simulink model "ACTUAL_REV3_TESTMETHOD"  (R2025b)
settings: Solver=FixedStepAuto  StartTime=0.0  StopTime=inf  RelTol=1e-3
undefined symbols (not defined in the file): IO397, Pull, pull, up
libraries: speedgoatlib_IO613 x3, speedgoatlib_fpga_analog_io x2, canmsglib x2, speedgoatlib_fpga x1
settings Model: Creator=liamb  LastModifiedBy=maxbr
settings SolverCC: ConcurrentTasks=on  PositivePriorityOrder=on
settings OptimizationCC: BlockReduction=off  OptimizeBlockIOStorage=off
settings DebuggingCC: TasksWithSamePriorityMsg=none
settings HardwareCC: ProdBitPerLong=64.0  ProdLongLongMode=on  ProdHWDeviceType=Intel->x86-64 (Linux 64)
settings RTWCC: SystemTargetFile=speedgoat.tlc  TemplateMakefile=slrealtime_default_tmf  Toolchain=Simulink Real-Time Toolchain  BuildConfiguration=Faster Runs  CodeExecutionProfiling=on  TargetLang=C++  Description=Speedgoat Real-Time Target Machine
settings SimulinkRealTimeTargetCC: SLRTFileLogMaxRuns=1.0  ExtModeMaxTrigDuration=10.0  ExtModeStaticAllocSize=1000000.0  ExtModeTransport=0.0  MultiwordLength=2048.0  DynamicStringBufferSize=256.0  PreserveMATLABNamespacesInGeneratedCode=on  SubcomponentCodeInterfacePackaging=Reusable function  MATLABClassNameForMDSCustomization=Simulink.SoftwareTarget.GRTCustomization  InstructionSetFMA=off  LogToMDFFile=off

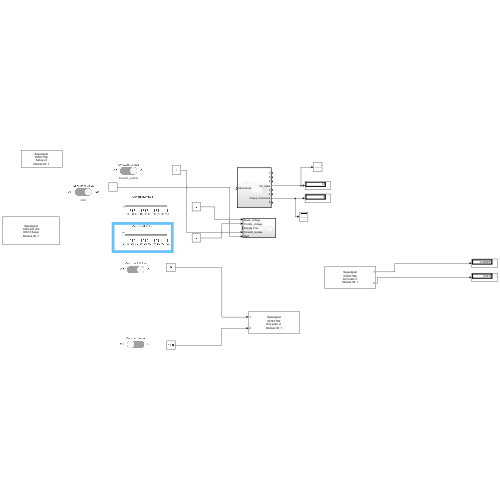
[thumbnail: Simulink's stored preview of the top-level diagram]
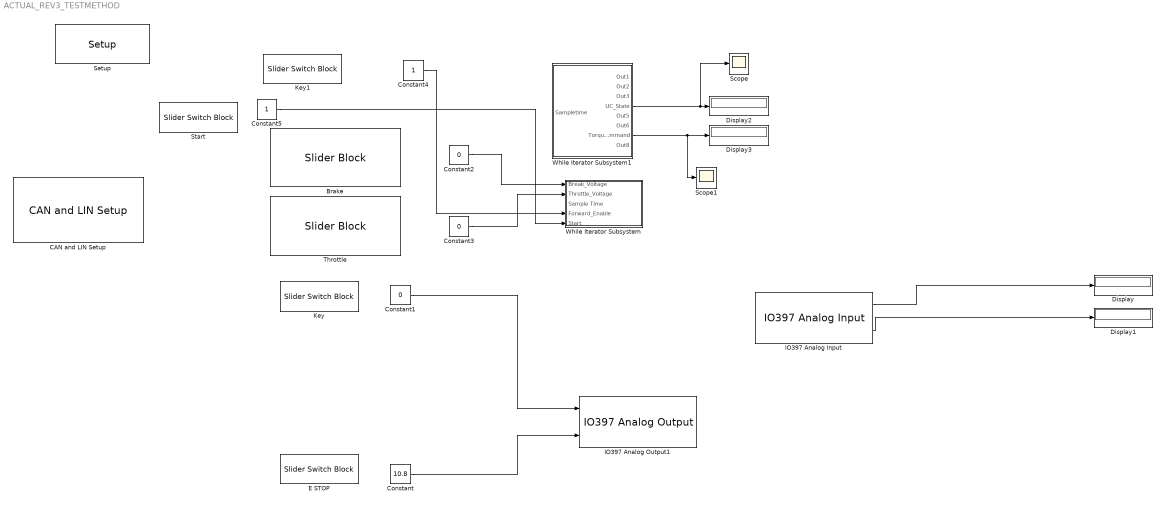
== system ACTUAL_REV3_TESTMETHOD ==
  Brake : SliderBlock
  "CAN and LIN Setup " : speedgoatlib_IO613/CAN and LIN Setup   moduleInitValues="[613    1    1   -1   -1]"  id=1  moduleType=IO613  pciSlot=-1  canChn1=CAN (HS)  canChn2=CAN (HS)  canChn3=Disabled  canChn4=Disabled  linChn1=Disabled  linChn2=Disabled  canInitStructArray=[]  canTermStructArray=[]  canChn1InitValues="[2   4   1  31   8   2   1  15   4]"  arbBdrChn1=500 kBaud  arbManBdrChn1=[4,1,31,8]  fdBdrChn1=2.0 MBaud  fdManBdrChn1=[2,1,15,4]  canChn2InitValues="[2   4   1  31   8   2   1  15   4]"  arbBdrChn2=500 kBaud  arbManBdrChn2=[4,1,31,8]  fdBdrChn2=2.0 MBaud  fdManBdrChn2=[2,1,15,4]  canChn3InitValues="[1   2   1  31   8   2   1   5   2]"  arbBdrChn3=1.0 MBaud  arbManBdrChn3=[2,1,31,8]  fdBdrChn3=5.0 MBaud  fdManBdrChn3=[2,1,5,2]  canChn4InitValues="[1   2   1  31   8   2   1   5   2]"  arbBdrChn4=1.0 MBaud  arbManBdrChn4=[2,1,31,8]  fdBdrChn4=5.0 MBaud  fdManBdrChn4=[2,1,5,2]  bdrLIN1=19200  linChn1InitValues="[1  19200]"  bdrLIN2=19200  linChn2InitValues="[1  19200]"
      settings: LibrarySourceBlock=speedgoatlib_CANLIN_OfA2/CAN and LIN Setup
  Constant : Constant  Value=10.8
  Constant1 : Constant  Value=0
  Constant2 : Constant  Value=0
  Constant3 : Constant  Value=0
  Constant4 : Constant
  Constant5 : Constant
  Display{,1..3} (4 alike) : Display
  E STOP : SliderSwitchBlock
  IO397 Analog Input : speedgoatlib_fpga_analog_io/IO397/IO397 Analog Input  openMaskCallback=0  id=1  chan=[1,2]  range=+5.12 V  parAiTriggerMode=I/O Module Clock  parAiInternalSignal=None  parAiDioTriggerChannel=1  parAiSampleRate=0  trigger=Initiator  ts=0.001
      settings: SourceProductName=Analog IO
  IO397 Analog Output1 : speedgoatlib_fpga_analog_io/IO397/IO397 Analog Output  id=1  chan=[1,2]  initVal=0  resetVal=0  ts=0.001  span=+-10.8 V
      settings: SourceProductName=Analog IO
  Key : SliderSwitchBlock
  Key1 : SliderSwitchBlock
      settings: AttributesFormatString=forward_enable
  Scope : Scope
      settings: ActiveDisplayYMinimum=-1  ActiveDisplayYMaximum=1
  Scope1 : Scope
      settings: ActiveDisplayYMinimum=-1  ActiveDisplayYMaximum=1
  Setup : speedgoatlib_fpga/Setup/Setup  board=IO397-50k  id=1  pciSlot=-1  device_id=1  bitstreamFilePath=C:\ProgramData\Speedgoat\bitstreams\io_configuration_package\R2025b\io397  bitstreamFile=speedgoat_IO397_HIL.mat  fpgaFreq=75000000  enableDma=off  rearEnb_1=off  rearIO_1=None  rearEnb_2=off  rearIO_2=None  ProgSpiFlash=off  ProgBPIFlash=off  useFpgaDmaController=off  dmaStopOnOverload=on  dmaModeSequential=on  dmaModeParallel=off  dmaTrigFixTime=on  dmaTrigA2B=off  dmaTriggerSourceSel=0  PullRPort15=pull-up 3.3V  PullRPort31=pull-up 3.3V  PullRPort47=pull-up 3.3V  PullRPort63=pull-up 3.3V  diffLineTermination_1=on  diffLineTermination_2=on  diffLineTermination_3=on  diffLineTermination_4=on  diffLineTermination_5=on  diffLineTermination_6=on  diffLineTermination_7=on  diffLineTermination_8=on  diffLineTermination_9=on  diffLineTermination_10=on  diffLineTermination_11=on  diffLineTermination_12=on  diffLineTermination_13=on  diffLineTermination_14=on  diffLineTermination_15=on  diffLineTermination_16=on  diffLineTermination_17=on  diffLineTermination_18=on  diffLineTermination_19=on  diffLineTermination_20=on  diffLineTermination_21=on  diffLineTermination_22=on  diffLineTermination_23=on  diffLineTermination_24=on  diffLineTermination_25=on  diffLineTermination_26=on  diffLineTermination_27=on  diffLineTermination_28=on  diffLineTermination_29=on  diffLineTermination_30=on  diffLineTermination_31=on  diffLineTermination_32=on  ioVoltageDropDown1=3.3V  pullResistorDropDown1_1=Pull-up  pullResistorDropDown1_2=Pull-up  pullResistorDropDown1_3=Pull-up  pullResistorDropDown1_4=Pull-up  pullResistorDropDown1_5=Pull-up  pullResistorDropDown1_6=Pull-up  pullResistorDropDown1_7=Pull-up  pullResistorDropDown1_8=Pull-up  ttlIsImplementedCheckBox1=off  pullResistorDropDown2=Pull-up  ioVoltageDropDown2=3.3V  ttlIsImplementedCheckBox2=off  pullResistorDropDown3=Pull-up  ioVoltageDropDown3=3.3V  ttlIsImplementedCheckBox3=off  pullResistorDropDown4=Pull-up  ioVoltageDropDown4=3.3V  ttlIsImplementedCheckBox4=off  pullResistorDropDown5=Pull-up  ioVoltageDropDown5=3.3V  ttlIsImplementedCheckBox5=off  pullResistorDropDown6=Pull-up  ioVoltageDropDown6=3.3V  ttlIsImplementedCheckBox6=off  pullResistorDropDown7=Pull-up  ioVoltageDropDown7=3.3V  ttlIsImplementedCheckBox7=off  pullResistorDropDown8=Pull-up  ioVoltageDropDown8=3.3V  ttlIsImplementedCheckBox8=off  terminationCheckBox1=off  terminationCheckBox2=off  terminationCheckBox3=off  terminationCheckBox4=off  diffIsImplementedCheckBox1=off  terminationCheckBox5=off  terminationCheckBox6=off  terminationCheckBox7=off  terminationCheckBox8=off  diffIsImplementedCheckBox2=off  terminationCheckBox9=off  terminationCheckBox10=off  terminationCheckBox11=off  terminationCheckBox12=off  diffIsImplementedCheckBox3=off  terminationCheckBox13=off  terminationCheckBox14=off  terminationCheckBox15=off  terminationCheckBox16=off  diffIsImplementedCheckBox4=off  terminationCheckBox17=off  terminationCheckBox18=off  terminationCheckBox19=off  terminationCheckBox20=off  diffIsImplementedCheckBox5=off  terminationCheckBox21=off  terminationCheckBox22=off  terminationCheckBox23=off  terminationCheckBox24=off  diffIsImplementedCheckBox6=off  terminationCheckBox25=off  terminationCheckBox26=off  terminationCheckBox27=off  terminationCheckBox28=off  diffIsImplementedCheckBox7=off  terminationCheckBox29=off  terminationCheckBox30=off  terminationCheckBox31=off  terminationCheckBox32=off  diffIsImplementedCheckBox8=off  PullRPort0_1=pull-up  VioPort0_1=3.3V  PullRPort1_1=pull-up  VioPort1_1=3.3V  PullRPort2_1=pull-up  VioPort2_1=3.3V  PullRPort3_1=pull-up  VioPort3_1=3.3V  PullRPort4_1=pull-up  VioPort4_1=3.3V  PullRPort5_1=pull-up  VioPort5_1=3.3V  PullRPort6_1=pull-up  VioPort6_1=3.3V  diffLineTermination_rear1_1=on  diffLineTermination_rear1_2=on  diffLineTermination_rear1_3=on  diffLineTermination_rear1_4=on  diffLineTermination_rear1_5=on  diffLineTermination_rear1_6=on  diffLineTermination_rear1_7=on  diffLineTermination_rear1_8=on  PullRPort0_2=pull-up  VioPort0_2=3.3V  PullRPort1_2=pull-up  VioPort1_2=3.3V  PullRPort2_2=pull-up  VioPort2_2=3.3V  PullRPort3_2=pull-up  VioPort3_2=3.3V  PullRPort4_2=pull-up  VioPort4_2=3.3V  PullRPort5_2=pull-up  VioPort5_2=3.3V  PullRPort6_2=pull-up  VioPort6_2=3.3V  diffLineTermination_rear2_1=on  diffLineTermination_rear2_2=on  diffLineTermination_rear2_3=on  diffLineTermination_rear2_4=on  diffLineTermination_rear2_5=on  diffLineTermination_rear2_6=on  diffLineTermination_rear2_7=on  diffLineTermination_rear2_8=on
      settings: SourceProductName=IO3xx
  Start : SliderSwitchBlock
      settings: AttributesFormatString=start
  Throttle : SliderBlock
  While Iterator Subsystem : Subsystem  TreatAsAtomicUnit=on
  While Iterator Subsystem1 : Subsystem  TreatAsAtomicUnit=on
  wires:
  Constant1/1 -> IO397 Analog Output1/1
  Constant3/1 -> While Iterator Subsystem/2(Throttle_Voltage)
  Constant2/1 -> While Iterator Subsystem/1(Break_Voltage)
  Constant/1 -> IO397 Analog Output1/2
  IO397 Analog Input/1 -> Display/1
  IO397 Analog Input/2 -> Display1/1
  While Iterator Subsystem1/7(Torque_Command) -> Scope1/1, Display3/1
  While Iterator Subsystem1/4(UC_State) -> Scope/1, Display2/1
  Constant4/1 -> While Iterator Subsystem/4(Forward_Enable)
  Constant5/1 -> While Iterator Subsystem/5(Start)

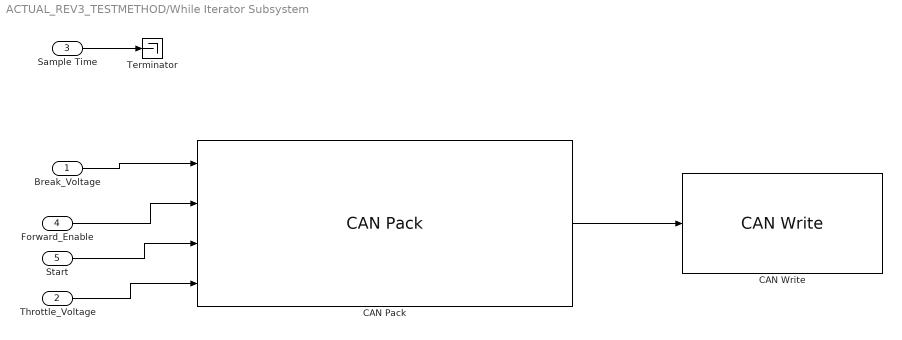
== system ACTUAL_REV3_TESTMETHOD/While Iterator Subsystem ==
  Break_Voltage : Inport
  Throttle_Voltage : Inport  Port=2
  Sample Time : Inport  Port=3
  Forward_Enable : Inport  Port=4
  Start : Inport  Port=5
  CAN Pack : canmsglib/CAN Pack  CANdbFile=C:\Users\maxbr\OneDrive\Documents\updatedpowertraindbcusethis.dbc  MsgList=Throttle_Position_and_Errors  MsgName=Throttle_Position_and_Errors  MsgIDType=Standard (11-bit identifier)  MsgIdentifier=208  CANIDInput=off  MsgLength=8  Remote=off  ApplyMinMax=off  BusOutput=off  SignalInfo={'Break_Voltage','16','16','LE','unsigned','Standard','0','1','0','0','65535';'Forward_Enable','48','1','LE','unsigned','Standard','0','1','0','0','1';'Start','49','1','LE','unsigned','Standard','0','1','0','0','1';'Throttle_Voltage','0','16','LE','unsigned','Standard','0','1','0','0','65535'}
      settings: DataFormat=CANdb specified signals
  "CAN Write " : speedgoatlib_IO613/CAN Write   moduleType=IO613  id=1  channel=1  canType=CAN (HS)  useBusIn=off  numOfMsg=1  enableInput=off  enableStatusPort=off  initValues=[613 1 0.01 0 1 1 0 1 0 0]  ts=.01
      settings: SourceProductName=IO613
  Terminator : Terminator
  wires:
  Break_Voltage/1 -> CAN Pack/1
  CAN Pack/1 -> "CAN Write "/1
  Sample Time/1 -> Terminator/1
  Forward_Enable/1 -> CAN Pack/2
  Throttle_Voltage/1 -> CAN Pack/4
  Start/1 -> CAN Pack/3

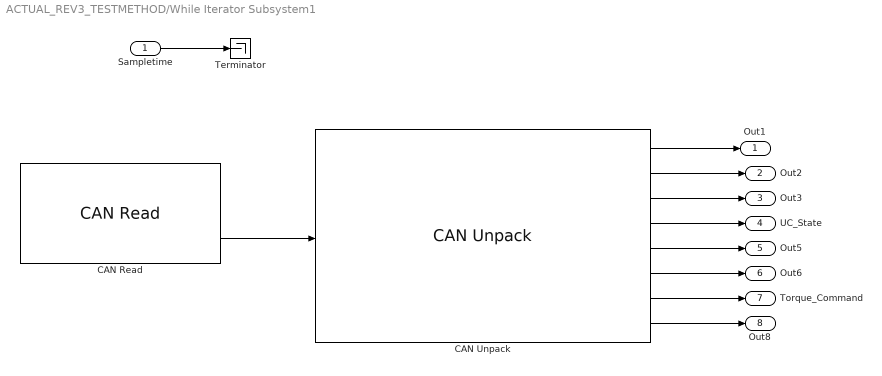
== system ACTUAL_REV3_TESTMETHOD/While Iterator Subsystem1 ==
  Sampletime : Inport
  "CAN Read " : speedgoatlib_IO613/CAN Read   moduleType=IO613  id=1  channel=1  canType=CAN (HS)  useBusOut=off  HasMulRead=Single Read from Buffer (FIFO)  MsgIDlist=[1 2]  isEFF=off  LabelInHex=on  enableInput=off  ts=.01  initValues=[613 1 0.01 0 1 1 0 0 0 1 2 1 2]
      settings: SourceProductName=IO613
  CAN Unpack : canmsglib/CAN Unpack  CANdbFile=C:\Users\maxbr\OneDrive\Documents\updatedpowertraindbcusethis.dbc  MsgList=M192_Command_Message  MsgName=M192_Command_Message  MsgIDType=Standard (11-bit identifier)  MsgIdentifier=192  MsgLength=8  SignalInfo={'VCU_INV_Direction_Command','32','1','LE','unsigned','Standard','0','1','0','0','1';'VCU_INV_Inverter_Discharge','41','1','LE','unsigned','Standard','0','1','0','0','1';'VCU_INV_Inverter_Enable','40','1','LE','unsigned','Standard','0','1','0','0','1';'VCU_INV_RollingCounter','44','4','LE','unsigned','Standard','0','1','0','0','15';'VCU_INV_Speed_Command','16','16','LE','signed','Standard','0','1','0','-32768','32767';'VCU_INV_Speed_Mode_Enable','42','1','LE','unsigned','Standard','0','1','0','0','1';'VCU_INV_Torque_Command','0','16','LE','signed','Standard','0','0.1','0','-3276.8','3276.7';'VCU_INV_Torque_Limit_Command','48','16','LE','signed','Standard','0','0.1','0','-3276.8','3276.7'}  IDPort=off  TimestampPort=off  ErrorPort=off  RemotePort=off  LengthPort=off  StatusPort=off  ApplyMinMax=off
      settings: DataFormat=CANdb specified signals
  Terminator : Terminator
  Out1 : Outport
  Out2 : Outport  Port=2
  Out3 : Outport  Port=3
  UC_State : Outport  Port=4
  Out5 : Outport  Port=5
  Out6 : Outport  Port=6
  Torque_Command : Outport  Port=7
  Out8 : Outport  Port=8
  wires:
  Sampletime/1 -> Terminator/1
  "CAN Read "/2 -> CAN Unpack/1
  CAN Unpack/8 -> Out8/1
  CAN Unpack/7 -> Torque_Command/1
  CAN Unpack/6 -> Out6/1
  CAN Unpack/5 -> Out5/1
  CAN Unpack/4 -> UC_State/1
  CAN Unpack/3 -> Out3/1
  CAN Unpack/2 -> Out2/1
  CAN Unpack/1 -> Out1/1
